simulink subsystem "Multisine_CZ1506"  (R2025a)
settings: Solver=VariableStepAuto  StartTime=0.0  StopTime=10.0  RelTol=1e-3
undefined symbols (not defined in the file): MS, MS2
settings Model: Creator=17036  LastModifiedBy=gurt1

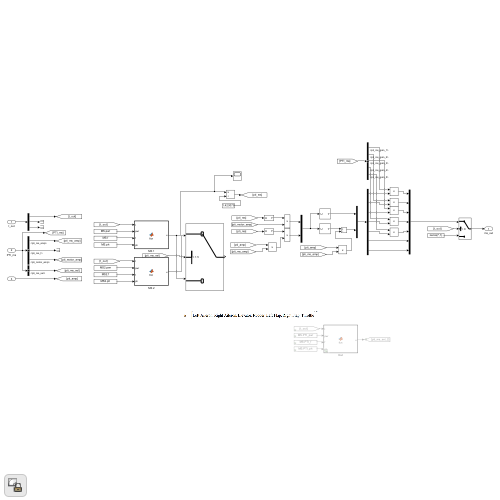
[thumbnail: Simulink's stored preview of the top-level diagram]
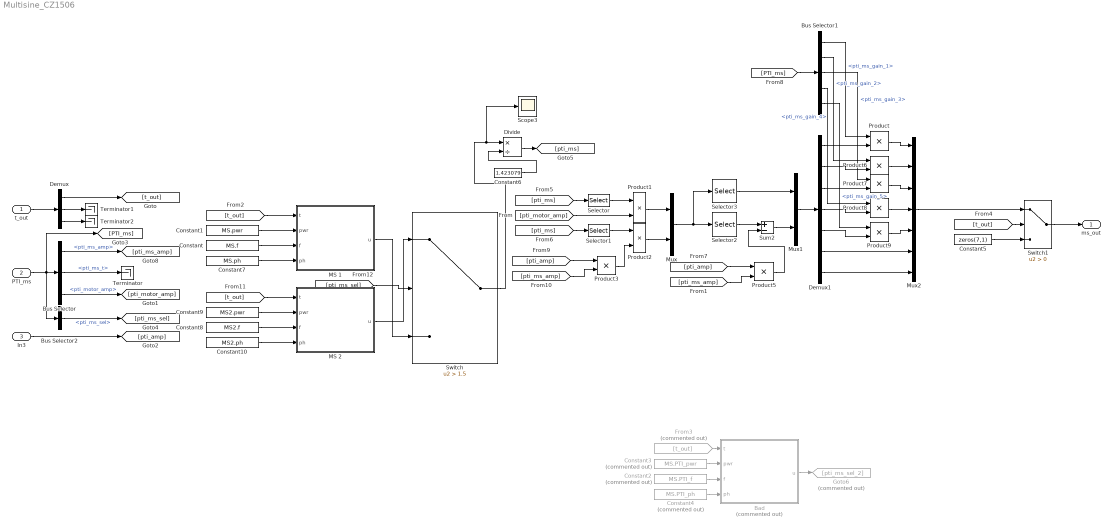
== system Multisine_CZ1506 ==
  t_out : Inport
  PTI_ms : Inport  Port=2
  In3 : Inport  Port=3
  Bad : MATLAB Function  Commented=on  TreatAsAtomicUnit=on
  Bus Selector : BusSelector  OutputSignals=pti_ms_amp,pti_ms_t,pti_motor_amp
  Bus Selector1 : BusSelector  OutputSignals=pti_ms_gain_1,pti_ms_gain_2,pti_ms_gain_3,pti_ms_gain_4,pti_ms_gain_5
  Bus Selector2 : BusSelector  OutputSignals=pti_ms_sel
  Constant : Constant  Value=MS.f
  Constant1 : Constant  Value=MS.pwr
  Constant10 : Constant  Value=MS2.ph
  Constant2 : Constant  Commented=on  Value=MS.PTI_f
  Constant3 : Constant  Commented=on  Value=MS.PTI_pwr
  Constant4 : Constant  Commented=on  Value=MS.PTI_ph
  Constant5 : Constant  Value=zeros(7,1)
  Constant6 : Constant  Value=1.423079  SampleTime=-1
  Constant7 : Constant  Value=MS.ph
  Constant8 : Constant  Value=MS2.f
  Constant9 : Constant  Value=MS2.pwr
  Demux : Demux  Outputs=3
  Demux1 : Demux  Outputs=7
  Divide : Product  Inputs=*/
  From3 : From  Commented=on  GotoTag=t_out
  Goto6 : Goto  Commented=on  GotoTag=pti_ms_sel_2
  MS 1 : MATLAB Function  TreatAsAtomicUnit=on
  MS 2 : MATLAB Function  TreatAsAtomicUnit=on
  Mux : Mux  Inputs=2
  Mux1 : Mux  Inputs=2
  Mux2 : Mux  Inputs=7
  Product{,1..3,5..9} (9 alike) : Product
  Scope3 : Scope
      settings: ActiveDisplayYMinimum=-2.51953125  ActiveDisplayYMaximum=1.2109375  DataLoggingVariableName=ScopeData8
  Selector : Selector  InputPortWidth=7  IndexOptions=Index vector (dialog)  Indices=7  OutputSizes=1
  Selector1 : Selector  InputPortWidth=7  IndexOptions=Index vector (dialog)  Indices=[1:6]  OutputSizes=1
  Selector2 : Selector  InputPortWidth=7  IndexOptions=Index vector (dialog)  Indices=[6,7]  OutputSizes=1
  Selector3 : Selector  InputPortWidth=7  IndexOptions=Index vector (dialog)  Indices=[1:5]  OutputSizes=1
  Sum2 : Sum  Inputs=+-
  Switch : Switch  Criteria=u2 > Threshold  Threshold=1.5  SaturateOnIntegerOverflow=off  InputSameDT=off
  Switch1 : Switch  Criteria=u2 > Threshold  SaturateOnIntegerOverflow=off  InputSameDT=off
  Terminator : Terminator
  Terminator1 : Terminator
  Terminator2 : Terminator
  ms_out : Outport
  wires:
  PTI_ms/1 -> Bus Selector/1, [PTI_ms], Bus Selector2/1
  Bus Selector/1 -> [pti_ms_amp]  "<pti_ms_amp>"
  Switch1/1 -> ms_out/1
  t_out/1 -> Demux/1
  Demux/2 -> Terminator1/1
  Bus Selector/2 -> Terminator/1  "<pti_ms_t>"
  Bad/1(u) -> Goto6/1
  Constant2/1 -> Bad/3(f)
  Constant4/1 -> Bad/4(ph)
  From3/1 -> Bad/1(t)
  Constant3/1 -> Bad/2(pwr)
  [t_out] -> Switch1/2
  Constant5/1 -> Switch1/3
  Demux/1 -> [t_out]
  Demux/3 -> Terminator2/1
  Bus Selector/3 -> [pti_motor_amp]  "<pti_motor_amp>"
  [pti_ms] -> Selector/1
  [pti_motor_amp] -> Product1/2
  Selector/1 -> Product1/1
  [pti_ms] -> Selector1/1
  Product1/1 -> Mux/1
  Selector1/1 -> Product2/1
  Product2/1 -> Mux/2
  Mux/1 -> Selector2/1, Selector3/1
  In3/1 -> [pti_amp]
  [t_out] -> MS 1/1(t)
  Constant1/1 -> MS 1/2(pwr)
  Constant/1 -> MS 1/3(f)
  Constant7/1 -> MS 1/4(ph)
  [pti_amp] -> Product3/1
  [pti_ms_amp] -> Product3/2
  Product3/1 -> Product2/2
  MS 1/1(u) -> Switch/3
  Selector2/1 -> Sum2/1
  Sum2/1 -> Mux1/2
  Selector3/1 -> Mux1/1
  Mux1/1 -> Demux1/1
  Product5/1 -> Sum2/2
  [pti_ms_amp] -> Product5/2
  [pti_amp] -> Product5/1
  Constant6/1 -> Divide/2
  Divide/1 -> [pti_ms]
  Demux1/6 -> Mux2/6
  Demux1/7 -> Mux2/7
  [PTI_ms] -> Bus Selector1/1
  Demux1/1 -> Product/2
  Product/1 -> Mux2/1
  Bus Selector1/1 -> Product/1  "<pti_ms_gain_1>"
  Product6/1 -> Mux2/2
  Bus Selector1/2 -> Product6/1  "<pti_ms_gain_2>"
  Demux1/2 -> Product6/2
  Product7/1 -> Mux2/3
  Bus Selector1/3 -> Product7/1  "<pti_ms_gain_3>"
  Demux1/3 -> Product7/2
  Product8/1 -> Mux2/4
  Demux1/4 -> Product8/2
  Bus Selector1/4 -> Product8/1  "<pti_ms_gain_4>"
  Product9/1 -> Mux2/5
  Demux1/5 -> Product9/2
  Bus Selector1/5 -> Product9/1  "<pti_ms_gain_5>"
  Mux2/1 -> Switch1/1
  Constant10/1 -> MS 2/4(ph)
  Constant8/1 -> MS 2/3(f)
  Constant9/1 -> MS 2/2(pwr)
  [t_out] -> MS 2/1(t)
  MS 2/1(u) -> Switch/1
  Bus Selector2/1 -> [pti_ms_sel]  "<pti_ms_sel>"
  [pti_ms_sel] -> Switch/2
  Switch/1 -> Divide/1, Scope3/1

== matlab function Multisine_CZ1506/MS 2 ==
  data: t input; u output; pwr input; f input; ph input
function u  = fcn(t,pwr,f,ph)

[nf,ni] = size(f);

u = zeros(ni,1);
t = double(t);

for jj=1:ni
    for kk = 1:nf
        u(jj) = u(jj)+sqrt(pwr(kk,jj))*sin(2*pi*f(kk,jj)*t+ph(kk,jj));
    end
end

== matlab function Multisine_CZ1506/Bad ==
  data: t input; u output; pwr input; f input; ph input
function u  = fcn(t,pwr,f,ph)

[nf,ni] = size(f);

u = zeros(ni,1);
t = double(t);

for jj=1:ni
    for kk = 1:nf
        u(jj) = u(jj)+sqrt(pwr(kk,jj))*sin(2*pi*f(kk,jj)*t+ph(kk,jj));
        %sin(2*pi*f(kk,jj)*t)
    end
end

== matlab function Multisine_CZ1506/MS 1 ==
  data: t input; u output; pwr input; f input; ph input
function u  = fcn(t,pwr,f,ph)

[nf,ni] = size(f);

u = zeros(ni,1);
t = double(t);

for jj=1:ni
    for kk = 1:nf
        u(jj) = u(jj)+sqrt(pwr(kk,jj))*sin(2*pi*f(kk,jj)*t+ph(kk,jj));
    end
end
